simulink model "scs3"  (R2017a)
settings: Solver=VariableStepAuto  StartTime=0.0  StopTime=100  RelTol=1e-3
libraries: xbsIndex_r4 x28, simulink x3
settings Model: Creator=vgssa  LastModifiedBy=vgssa

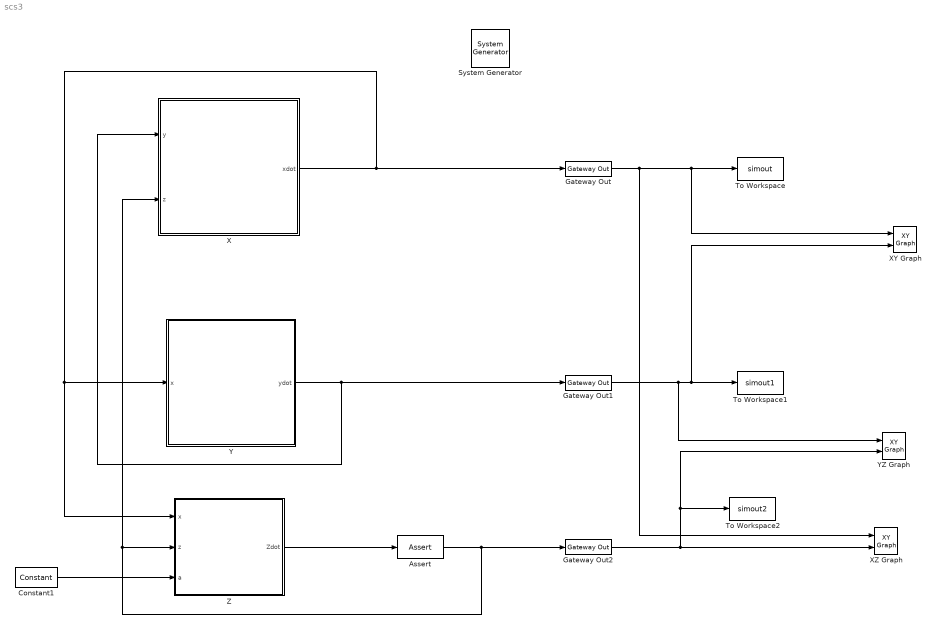
== system scs3 ==
  " System Generator" : xbsIndex_r4/ System Generator  Tag=genX  xilinxfamily=kintex7  part=xc7k325t  speed=-3  package=fbg676  synthesis_tool=Vivado  clock_wrapper=Clock Enables  directory=./netlist  proj_type=Vivado  Synth_file=Vivado Synthesis Defaults  Impl_file=Vivado Implementation Defaults  testbench=off  simulink_period=0.001  sysclk_period=10  dcm_input_clock_period=10  incr_netlist=off  trim_vbits=Everywhere in SubSystem  dbl_ovrd=According to Block Masks  core_generation=According to Block Masks  run_coregen=off  deprecated_control=off  eval_field=0  block_type=sysgen
  Assert : xbsIndex_r4/Assert  assert_type=on  type_source=Explicitly  gui_display_data_type=Fixed-point  arith_type="Signed  (2's comp)"  n_bits=32  bin_pt=16  preci_type=Single  exp_width=8  frac_width=24  assert_rate=on  rate_source=Explicitly  period=0.001  output_port=on  block_type=assert
      settings: block_version=12.2
  Constant1 : xbsIndex_r4/Constant  const=1  gui_display_data_type=Fixed-point  arith_type=Unsigned  n_bits=32  bin_pt=16  preci_type=Single  exp_width=8  frac_width=24  explicit_period=off  period=1  equ=P=C  opselect=C  inp2=PCIN>>17  opr=+  inp1=P  carry=CIN  dbl_ovrd=off  block_type=constant
  Gateway Out : xbsIndex_r4/Gateway Out  inherit_from_input=off  hdl_port=on  rows=1  columns=1  UseAsDAC=off  DACChannel='1'  interface=None  automatic_assignment=on  address_offset=hex2dec('00')  intf_name=''  intf_description=''  timing_constraint=None  locs_specified=off  LOCs={}  io_standard={}  block_type=gatewayout
      settings: infoedit="Gateway out block.  Converts Xilinx fixed point inputs into ouputs of type Simulink integer, double, or fixed point.<br><br>Hardware notes:  In hardware these blocks become top level output ports or are discarded, depending on how they are configured."  block_version=12.2
  Gateway Out1 : xbsIndex_r4/Gateway Out  inherit_from_input=off  hdl_port=on  rows=1  columns=1  UseAsDAC=off  DACChannel='1'  interface=None  automatic_assignment=on  address_offset=hex2dec('00')  intf_name=''  intf_description=''  timing_constraint=None  locs_specified=off  LOCs={}  io_standard={}  block_type=gatewayout
      settings: infoedit="Gateway out block.  Converts Xilinx fixed point inputs into ouputs of type Simulink integer, double, or fixed point.<br><br>Hardware notes:  In hardware these blocks become top level output ports or are discarded, depending on how they are configured."  block_version=12.2
  Gateway Out2 : xbsIndex_r4/Gateway Out  inherit_from_input=off  hdl_port=on  rows=1  columns=1  UseAsDAC=off  DACChannel='1'  interface=None  automatic_assignment=on  address_offset=hex2dec('00')  intf_name=''  intf_description=''  timing_constraint=None  locs_specified=off  LOCs={}  io_standard={}  block_type=gatewayout
      settings: infoedit="Gateway out block.  Converts Xilinx fixed point inputs into ouputs of type Simulink integer, double, or fixed point.<br><br>Hardware notes:  In hardware these blocks become top level output ports or are discarded, depending on how they are configured."  block_version=12.2
  To Workspace : ToWorkspace  VariableName=simout  SaveFormat=Structure  SampleTime=-1
  To Workspace1 : ToWorkspace  VariableName=simout1  SaveFormat=Structure  SampleTime=-1
  To Workspace2 : ToWorkspace  VariableName=simout2  SaveFormat=Structure  SampleTime=-1
  X : Subsystem
  XY Graph : simulink/Sinks/XY Graph  xmin=-1  xmax=1  ymin=-1  ymax=1  st=-1
  XZ Graph : simulink/Sinks/XY Graph  xmin=-1  xmax=1  ymin=-1  ymax=1  st=-1
  Y : Subsystem
  YZ Graph : simulink/Sinks/XY Graph  xmin=-1  xmax=1  ymin=-1  ymax=1  st=-1
  Z : Subsystem
  wires:
  Z/1(Zdot) -> Assert/1
  Gateway Out/1 -> XZ Graph/1, XY Graph/1, To Workspace/1
  X/1(xdot) -> Y/1("x "), Z/1("x "), Gateway Out/1
  Gateway Out1/1 -> YZ Graph/1, XY Graph/2, To Workspace1/1
  Y/1(ydot) -> X/1(y), Gateway Out1/1
  Assert/1 -> Z/2("z "), X/2(z), Gateway Out2/1
  Gateway Out2/1 -> XZ Graph/2, YZ Graph/2, To Workspace2/1
  Constant1/1 -> Z/3(a)

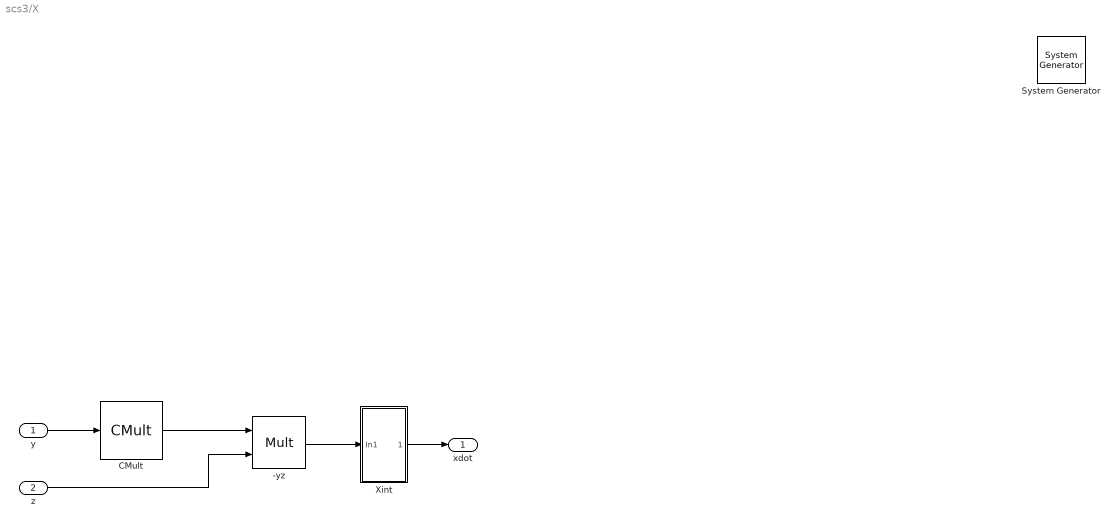
== system scs3/X ==
  y : Inport
  z : Inport  Port=2
  " System Generator" : xbsIndex_r4/ System Generator  Tag=genX  xilinxfamily=Kintex7  part=xc7k325t  speed=-3  package=fbg676  synthesis_tool=Vivado  clock_wrapper=Clock Enables  directory=./netlist  proj_type=Vivado  Synth_file=Vivado Synthesis Defaults  Impl_file=Vivado Implementation Defaults  testbench=off  simulink_period=1  sysclk_period=10  dcm_input_clock_period=10  incr_netlist=off  trim_vbits=Everywhere in SubSystem  dbl_ovrd=According to Block Masks  core_generation=According to Block Masks  run_coregen=off  deprecated_control=off  eval_field=0  block_type=sysgen
  -yz : xbsIndex_r4/Mult  precision=Full  arith_type="Signed  (2's comp)"  n_bits=16  bin_pt=14  quantization=Truncate  overflow=Wrap  en=off  latency=0  use_behavioral_HDL=off  opt=Speed  use_embedded=on  optimum_pipeline=off  pipeline=on  dbl_ovrd=off  use_rpm=on  placement_style=Triangular  block_type=mult
  CMult : xbsIndex_r4/CMult  const=-1  gui_display_data_type=Fixed-point  const_n_bits=32  const_bin_pt=16  float_type=Single  exp_bits=8  fraction_bits=24  en=off  latency=0  precision=Full  arith_type="Signed  (2's comp)"  n_bits=16  bin_pt=14  quantization=Truncate  overflow=Wrap  use_behavioral_HDL=off  mem_type=Distributed RAM  pipeline=off  dbl_ovrd=off  block_type=cmult
  Xint : Subsystem
  xdot : Outport
  wires:
  Xint/1(Out1) -> xdot/1
  z/1 -> -yz/2
  y/1 -> CMult/1
  CMult/1 -> -yz/1
  -yz/1 -> Xint/1(In1)

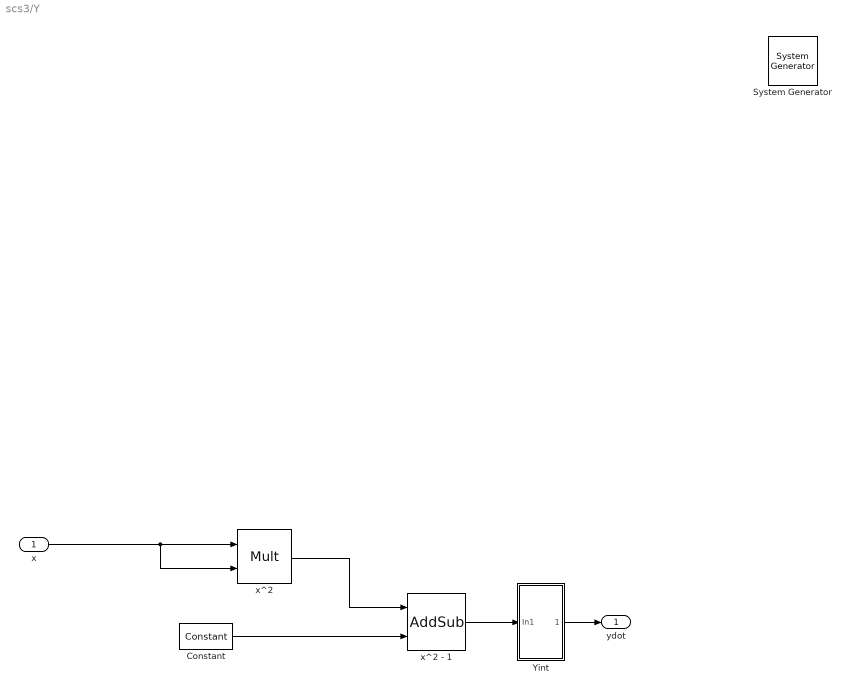
== system scs3/Y ==
  "x " : Inport
  " System Generator" : xbsIndex_r4/ System Generator  Tag=genX  xilinxfamily=Kintex7  part=xc7k325t  speed=-3  package=fbg676  synthesis_tool=Vivado  clock_wrapper=Clock Enables  directory=./netlist  proj_type=Vivado  Synth_file=Vivado Synthesis Defaults  Impl_file=Vivado Implementation Defaults  testbench=off  simulink_period=1  sysclk_period=10  dcm_input_clock_period=10  incr_netlist=off  trim_vbits=Everywhere in SubSystem  dbl_ovrd=According to Block Masks  core_generation=According to Block Masks  run_coregen=off  deprecated_control=off  eval_field=0  block_type=sysgen
  Constant : xbsIndex_r4/Constant  const=1  gui_display_data_type=Fixed-point  arith_type=Unsigned  n_bits=32  bin_pt=16  preci_type=Single  exp_width=8  frac_width=24  explicit_period=off  period=1  equ=P=C  opselect=C  inp2=PCIN>>17  opr=+  inp1=P  carry=CIN  dbl_ovrd=off  block_type=constant
  Yint : Subsystem
  x^2 : xbsIndex_r4/Mult  precision=Full  arith_type="Signed  (2's comp)"  n_bits=16  bin_pt=14  quantization=Truncate  overflow=Wrap  en=off  latency=0  use_behavioral_HDL=off  opt=Speed  use_embedded=on  optimum_pipeline=off  pipeline=on  dbl_ovrd=off  use_rpm=on  placement_style=Triangular  block_type=mult
  x^2 - 1 : xbsIndex_r4/AddSub  mode=Subtraction  use_carryin=off  use_carryout=off  en=off  latency=0  precision=Full  arith_type=Unsigned  n_bits=16  bin_pt=14  quantization=Truncate  overflow=Wrap  use_behavioral_HDL=off  hw_selection=Fabric  pipelined=off  dbl_ovrd=off  block_type=addsub
  ydot : Outport
  wires:
  Yint/1(Out1) -> ydot/1
  "x "/1 -> x^2/2, x^2/1
  x^2/1 -> x^2 - 1/1
  Constant/1 -> x^2 - 1/2
  x^2 - 1/1 -> Yint/1(In1)

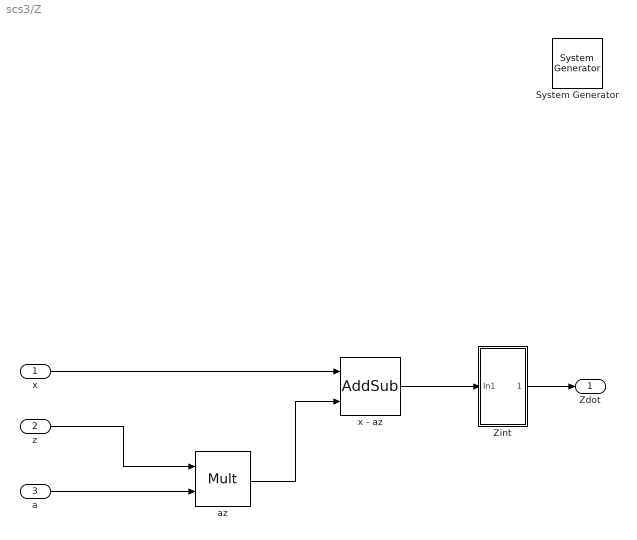
== system scs3/Z ==
  "x " : Inport
  "z " : Inport  Port=2
  a : Inport  Port=3
  " System Generator" : xbsIndex_r4/ System Generator  Tag=genX  xilinxfamily=Kintex7  part=xc7k325t  speed=-3  package=fbg676  synthesis_tool=Vivado  clock_wrapper=Clock Enables  directory=./netlist  proj_type=Vivado  Synth_file=Vivado Synthesis Defaults  Impl_file=Vivado Implementation Defaults  testbench=off  simulink_period=1  sysclk_period=10  dcm_input_clock_period=10  incr_netlist=off  trim_vbits=Everywhere in SubSystem  dbl_ovrd=According to Block Masks  core_generation=According to Block Masks  run_coregen=off  deprecated_control=off  eval_field=0  block_type=sysgen
  Zint : Subsystem
  az : xbsIndex_r4/Mult  precision=Full  arith_type="Signed  (2's comp)"  n_bits=16  bin_pt=14  quantization=Truncate  overflow=Wrap  en=off  latency=0  use_behavioral_HDL=off  opt=Speed  use_embedded=on  optimum_pipeline=off  pipeline=on  dbl_ovrd=off  use_rpm=on  placement_style=Triangular  block_type=mult
  x - az : xbsIndex_r4/AddSub  mode=Subtraction  use_carryin=off  use_carryout=off  en=off  latency=0  precision=Full  arith_type=Unsigned  n_bits=16  bin_pt=14  quantization=Truncate  overflow=Wrap  use_behavioral_HDL=off  hw_selection=Fabric  pipelined=off  dbl_ovrd=off  block_type=addsub
  Zdot : Outport
  wires:
  Zint/1(Out1) -> Zdot/1
  "z "/1 -> az/1
  a/1 -> az/2
  az/1 -> x - az/2
  "x "/1 -> x - az/1
  x - az/1 -> Zint/1(In1)

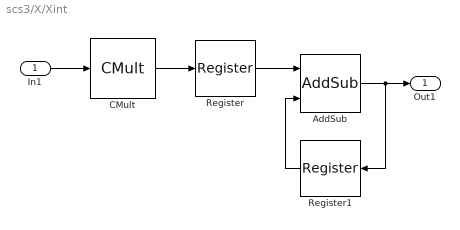
== system scs3/X/Xint ==
  In1 : Inport
  AddSub : xbsIndex_r4/AddSub  mode=Addition  use_carryin=off  use_carryout=off  en=off  latency=0  precision=User Defined  arith_type="Signed  (2's comp)"  n_bits=32  bin_pt=16  quantization="Round  (unbiased: +/- Inf)"  overflow=Wrap  use_behavioral_HDL=off  hw_selection=Fabric  pipelined=off  dbl_ovrd=off  block_type=addsub
      settings: block_version=12.2
  CMult : xbsIndex_r4/CMult  const=0.001007  gui_display_data_type=Fixed-point  const_n_bits=32  const_bin_pt=16  float_type=Single  exp_bits=8  fraction_bits=24  en=off  latency=0  precision=User Defined  arith_type="Signed  (2's comp)"  n_bits=32  bin_pt=16  quantization="Round  (unbiased: +/- Inf)"  overflow=Wrap  use_behavioral_HDL=off  mem_type=Distributed RAM  pipeline=off  dbl_ovrd=off  block_type=cmult
      settings: block_version=12.2
  Register : xbsIndex_r4/Register  init=1  rst=off  en=off  dbl_ovrd=off  block_type=register
      settings: block_version=12.2
  Register1 : xbsIndex_r4/Register  init=0  rst=off  en=off  dbl_ovrd=off  block_type=register
      settings: block_version=12.2
  Out1 : Outport
  wires:
  CMult/1 -> Register/1
  Register/1 -> AddSub/1
  AddSub/1 -> Register1/1, Out1/1
  Register1/1 -> AddSub/2
  In1/1 -> CMult/1

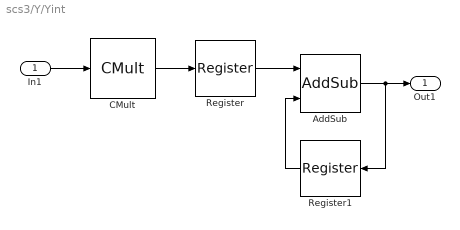
== system scs3/Y/Yint ==
  In1 : Inport
  AddSub : xbsIndex_r4/AddSub  mode=Addition  use_carryin=off  use_carryout=off  en=off  latency=0  precision=User Defined  arith_type="Signed  (2's comp)"  n_bits=32  bin_pt=16  quantization="Round  (unbiased: +/- Inf)"  overflow=Wrap  use_behavioral_HDL=off  hw_selection=Fabric  pipelined=off  dbl_ovrd=off  block_type=addsub
      settings: block_version=12.2
  CMult : xbsIndex_r4/CMult  const=0.001007  gui_display_data_type=Fixed-point  const_n_bits=32  const_bin_pt=16  float_type=Single  exp_bits=8  fraction_bits=24  en=off  latency=0  precision=User Defined  arith_type="Signed  (2's comp)"  n_bits=32  bin_pt=16  quantization="Round  (unbiased: +/- Inf)"  overflow=Wrap  use_behavioral_HDL=off  mem_type=Distributed RAM  pipeline=off  dbl_ovrd=off  block_type=cmult
      settings: block_version=12.2
  Register : xbsIndex_r4/Register  init=1  rst=off  en=off  dbl_ovrd=off  block_type=register
      settings: block_version=12.2
  Register1 : xbsIndex_r4/Register  init=0  rst=off  en=off  dbl_ovrd=off  block_type=register
      settings: block_version=12.2
  Out1 : Outport
  wires:
  CMult/1 -> Register/1
  Register/1 -> AddSub/1
  AddSub/1 -> Register1/1, Out1/1
  Register1/1 -> AddSub/2
  In1/1 -> CMult/1

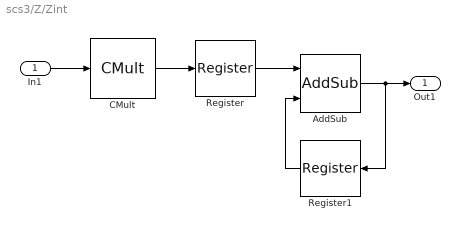
== system scs3/Z/Zint ==
  In1 : Inport
  AddSub : xbsIndex_r4/AddSub  mode=Addition  use_carryin=off  use_carryout=off  en=off  latency=0  precision=User Defined  arith_type="Signed  (2's comp)"  n_bits=32  bin_pt=16  quantization="Round  (unbiased: +/- Inf)"  overflow=Wrap  use_behavioral_HDL=off  hw_selection=Fabric  pipelined=off  dbl_ovrd=off  block_type=addsub
      settings: block_version=12.2
  CMult : xbsIndex_r4/CMult  const=0.001007  gui_display_data_type=Fixed-point  const_n_bits=32  const_bin_pt=16  float_type=Single  exp_bits=8  fraction_bits=24  en=off  latency=0  precision=User Defined  arith_type="Signed  (2's comp)"  n_bits=32  bin_pt=16  quantization="Round  (unbiased: +/- Inf)"  overflow=Wrap  use_behavioral_HDL=off  mem_type=Distributed RAM  pipeline=off  dbl_ovrd=off  block_type=cmult
      settings: block_version=12.2
  Register : xbsIndex_r4/Register  init=-1  rst=off  en=off  dbl_ovrd=off  block_type=register
      settings: block_version=12.2
  Register1 : xbsIndex_r4/Register  init=0  rst=off  en=off  dbl_ovrd=off  block_type=register
      settings: block_version=12.2
  Out1 : Outport
  wires:
  CMult/1 -> Register/1
  Register/1 -> AddSub/1
  AddSub/1 -> Register1/1, Out1/1
  Register1/1 -> AddSub/2
  In1/1 -> CMult/1
